simulink model "ramadan_2021"  (R2020a)
settings: Solver=ode15s  StartTime=0.0  StopTime=20  MaxStep=1e-2  MinStep=1e-20  RelTol=1e-3
StartFcn:
  | tic
StopFcn:
  | toc
  | 
  | 
  | %if GimbalLockFlag
  |  % fprintf(2, 'Almost reached Gimbal Lock of IMU. Simulation stopped.\n')
  | %end
  | 
  | %fprintf('Elapsed time: %4.2f sec (%4.2f%% realtime)\n', a, tout(end)/a*100)
values from neighbouring files (symbols this model uses):
  Balance02 = param(28:31)    [assign_parameters.m]
  Balance13 = param(32:35)    [assign_parameters.m]
  BalanceTrunk = param(22:23)    [assign_parameters.m]
  BalanceTrunkLat = param(24:27)    [assign_parameters.m]
  BasisStim = param(1:11)    [assign_parameters.m]
  CompliantLeg = param(12:14)    [assign_parameters.m]
  CompliantLegLat = param(15)    [assign_parameters.m]
  PreventKneeOverextension = param(16:21)    [assign_parameters.m]
  propulsion = dataset(i,3)    [AssignDataset_BasisPoints.m]    (also in assign_parameters.m = param(43))
  stepDur = dataset(i,2)    [AssignDataset_BasisPoints.m]    (also in assign_parameters.m = param(44))
  Target02 = dataset(i,8:10)    [AssignDataset_BasisPoints.m]    (also in assign_parameters.m = param(36:38))
  Target13 = dataset(i,5:7)    [AssignDataset_BasisPoints.m]    (also in assign_parameters.m = param(39:41))
  Target_lat = param(45)    [assign_parameters.m]
  theta0 = dataset(i,4)    [AssignDataset_BasisPoints.m]    (also in assign_parameters.m = param(42))
  v_init = dataset(i,1)    [AssignDataset_BasisPoints.m]    (also in assign_parameters.m = 1.25)
  WramameiSL_1000 = readmatrix('WSL_1000_Norm_Sigmoid_MSE_cont.csv')    [nms3D_prep.m]
  ZramameiSL_1000 = readmatrix('ZSL_1000_Norm_Sigmoid_MSE_cont.csv')    [nms3D_prep.m]
undefined symbols (not defined in the file or in its folder): ICs, mParams, X, Y, Z
libraries: nesl_utility x110, sm_lib x88, simulink x81, eeGeneralControl x30, robotmaniplib x10, dspinverses x9, robotcorelib x5, dspmathops x3, vrlib x1
(part 5 of 8)

== system ramadan_2021/Body and Contact Model/R Leg/Sensor Right Ankle ==
  note: Position and Velocity Sensor in World Frame
  Frame Sensor : sm_lib/Frames and Transforms/Transform Sensor  MeasurementFrame=Base  SenseAngle=off  SenseAxis=off  SenseAngle1=off  SenseAngle2=off  SenseAngle3=off  SenseQ=off  SenseR=off  SenseOmegaX=off  SenseOmegaY=off  SenseOmegaZ=off  SenseOmega1=off  SenseOmega2=off  SenseOmega3=off  SenseQDot=off  SenseRDot=off  SenseAlphaX=off  SenseAlphaY=off  SenseAlphaZ=off  SenseAlpha1=off  SenseAlpha2=off  SenseAlpha3=off  SenseQDDot=off  SenseRDDot=off  SenseX=on  SenseY=on  SenseZ=on  SenseRad=off  SenseAzim=off  SenseDist=off  SenseInc=off  SenseXDot=on  SenseYDot=on  SenseZDot=on  SenseRadDot=off  SenseAzimDot=off  SenseDistDot=off  SenseIncDot=off  SenseXDDot=off  SenseYDDot=off  SenseZDDot=off  SenseRadDDot=off  SenseAzimDDot=off  SenseDistDDot=off  SenseIncDDot=off
  Mux : Mux  Inputs=3
  Mux1 : Mux  Inputs=3
  PS-Simulink Converter1 : nesl_utility/PS-Simulink Converter  PhysicalDomain=network_engine_domain  SubClassName=ps_output  LeftPortType=input  RightPortType=output  PseudoPeriodic=off  Frequencies=[]  Unit=m  AffineConversion=off
  PS-Simulink Converter12 : nesl_utility/PS-Simulink Converter  PhysicalDomain=network_engine_domain  SubClassName=ps_output  LeftPortType=input  RightPortType=output  PseudoPeriodic=off  Frequencies=[]  Unit=m  AffineConversion=off
  PS-Simulink Converter2 : nesl_utility/PS-Simulink Converter  PhysicalDomain=network_engine_domain  SubClassName=ps_output  LeftPortType=input  RightPortType=output  PseudoPeriodic=off  Frequencies=[]  Unit=m  AffineConversion=off
  PS-Simulink Converter3 : nesl_utility/PS-Simulink Converter  PhysicalDomain=network_engine_domain  SubClassName=ps_output  LeftPortType=input  RightPortType=output  PseudoPeriodic=off  Frequencies=[]  Unit=m/s  AffineConversion=off
  PS-Simulink Converter4 : nesl_utility/PS-Simulink Converter  PhysicalDomain=network_engine_domain  SubClassName=ps_output  LeftPortType=input  RightPortType=output  PseudoPeriodic=off  Frequencies=[]  Unit=m/s  AffineConversion=off
  PS-Simulink Converter5 : nesl_utility/PS-Simulink Converter  PhysicalDomain=network_engine_domain  SubClassName=ps_output  LeftPortType=input  RightPortType=output  PseudoPeriodic=off  Frequencies=[]  Unit=m/s  AffineConversion=off
  World Frame : sm_lib/Frames and Transforms/World Frame
  Frame : PMIOPort  Side=Left
  Position [m] : Outport  VectorParamsAs1DForOutWhenUnconnected=off
  Velocity [m/s] : Outport  Port=2  VectorParamsAs1DForOutWhenUnconnected=off
  wires:
  PS-Simulink Converter12/1 -> Mux/1
  PS-Simulink Converter1/1 -> Mux/2
  PS-Simulink Converter2/1 -> Mux/3
  Mux/1 -> Position [m]/1
  PS-Simulink Converter5/1 -> Mux1/3
  PS-Simulink Converter4/1 -> Mux1/1
  Mux1/1 -> Velocity [m/s]/1
  PS-Simulink Converter3/1 -> Mux1/2
  connections:
  Frame Sensor/RConn1 -- Frame/RConn1
  PS-Simulink Converter12/LConn1 -- Frame Sensor/RConn2
  Frame Sensor/RConn3 -- PS-Simulink Converter1/LConn1
  Frame Sensor/RConn4 -- PS-Simulink Converter2/LConn1
  Frame Sensor/RConn7 -- PS-Simulink Converter5/LConn1
  Frame Sensor/RConn5 -- PS-Simulink Converter4/LConn1
  Frame Sensor/RConn6 -- PS-Simulink Converter3/LConn1
  World Frame/RConn1 -- Frame Sensor/LConn1

== system ramadan_2021/Body and Contact Model/R Leg/Shank ==
  Solid : sm_lib/Body Elements/Brick Solid  GraphicAmbientColor=[0.15 0.15 0.15 1.0]  BasedOnType=Density  BrickDimensions="[mParams.bodies.shank.d  mParams.bodies.shank.l mParams.bodies.shank.b]"  BrickDimensionUnits=m  CenterOfMass=mParams.bodies.shank.CG  CenterOfMassUnits=m  GraphicDiffuseColor=[1 0.5 0.5]  Density=2.7  DensityUnits=g/cm^3  DoExposeReferenceFrame=on  GraphicEmissiveColor=[0 0 0 1.0]  ExportEntireGeometry=off  SerializedFrames=<Frames><Frame><Id>Frame1</Id><Value><Name>F1</Name><Origin><Source>CenterOfMassFrame</Source><FeatureName></FeatureName></Origin><PrimaryAxis><DefinedDirection>+Z</DefinedDirection><Source>ReferenceFrame</Source><SourceDirection>+Z</SourceDirection><FeatureName></FeatureName></PrimaryAxis><SecondaryAxis><DefinedDirection>+X</DefinedDirection><Source>ReferenceFrame</Source><SourceDirection>+X</SourceDirection><FeatureName></FeatureName></SecondaryAxis></Value></Frame></Frames>  MarkerShape=Sphere  MarkerSize=10  GraphicType=FromGeometry  InertiaType=Custom  Mass=mParams.bodies.shank.m  MassUnits=kg  MomentsOfInertia=mParams.bodies.shank.In  MomentsOfInertiaUnits=kg*m^2  GraphicOpacity=1.0  ProductsOfInertia=[0 0 0]  ProductsOfInertiaUnits=kg*m^2  GraphicShininess=75  GraphicSpecularColor=[0.5 0.5 0.5 1.0]  GraphicVisPropType=SimpleVisualProperties
  Transform CS1 to MidSegment : sm_lib/Frames and Transforms/Rigid Transform  TranslationMethod=Cartesian  TranslationStandardOffset=0  TranslationLengthUnit=m  TranslationStandardAxis=+Y  TranslationCartesianOffset=[0 -mParams.bodies.shank.l/2 0]  TranslationROffset=0  TranslationROffsetUnits=m  TranslationZOffset=0  TranslationZOffsetUnits=m  TranslationThetaOffset=0  TranslationThetaOffsetUnits=deg  RotationMethod=None  RotationAngleUnits=deg  RotationStandardAxis=+X  RotationAngle=-90  RotationArbitraryAxis=[0 0 1]  FollAlignAxisA=+X  BaseAlignAxisA=+Y  FollAlignAxisB=+Y  BaseAlignAxisB=+Z  RotationSequenceAxes=FollowerAxes  RotationSequence=XYX  RotationSequenceAngles=[0 0 0]  RotationSequenceAnglesUnits=deg  RotationMatrix=[1 0 0; 0 1 0; 0 0 1]
  Transform MidSegment to CS2 : sm_lib/Frames and Transforms/Rigid Transform  TranslationMethod=Cartesian  TranslationStandardOffset=0  TranslationLengthUnit=m  TranslationStandardAxis=+Y  TranslationCartesianOffset=[ 0 -mParams.bodies.shank.l/2 0]  TranslationROffset=0  TranslationROffsetUnits=m  TranslationZOffset=0  TranslationZOffsetUnits=m  TranslationThetaOffset=0  TranslationThetaOffsetUnits=deg  RotationMethod=None  RotationAngleUnits=deg  RotationStandardAxis=+X  RotationAngle=90  RotationArbitraryAxis=[0 0 1]  FollAlignAxisA=+X  BaseAlignAxisA=+Y  FollAlignAxisB=+Y  BaseAlignAxisB=+Z  RotationSequenceAxes=FollowerAxes  RotationSequence=XYX  RotationSequenceAngles=[0 0 0]  RotationSequenceAnglesUnits=deg  RotationMatrix=[1 0 0; 0 1 0; 0 0 1]
  CS1 : PMIOPort  Side=Left
  CS2 : PMIOPort  Port=2  Side=Right
  connections:
  Transform MidSegment to CS2/LConn1 -- Transform CS1 to MidSegment/RConn1 -- Solid/RConn1
  Transform CS1 to MidSegment/LConn1 -- CS1/RConn1
  Transform MidSegment to CS2/RConn1 -- CS2/RConn1

== system ramadan_2021/Body and Contact Model/R Leg/Thigh ==
  Solid1 : sm_lib/Body Elements/Brick Solid  GraphicAmbientColor=[0.15 0.15 0.15 1.0]  BasedOnType=Density  BrickDimensions=[mParams.bodies.thigh.d mParams.bodies.thigh.l mParams.bodies.thigh.b]  BrickDimensionUnits=m  CenterOfMass=mParams.bodies.thigh.CG  CenterOfMassUnits=m  GraphicDiffuseColor=[1 0.5 0.5]  Density=2.7  DensityUnits=g/cm^3  DoExposeReferenceFrame=on  GraphicEmissiveColor=[0 0 0 1.0]  ExportEntireGeometry=off  SerializedFrames=<Frames><Frame><Id>Frame1</Id><Value><Name>F1</Name><Origin><Source>CenterOfMassFrame</Source><FeatureName></FeatureName></Origin><PrimaryAxis><DefinedDirection>+Z</DefinedDirection><Source>ReferenceFrame</Source><SourceDirection>+Z</SourceDirection><FeatureName></FeatureName></PrimaryAxis><SecondaryAxis><DefinedDirection>+X</DefinedDirection><Source>ReferenceFrame</Source><SourceDirection>+X</SourceDirection><FeatureName></FeatureName></SecondaryAxis></Value></Frame></Frames>  MarkerShape=Sphere  MarkerSize=10  GraphicType=FromGeometry  InertiaType=Custom  Mass=mParams.bodies.thigh.m  MassUnits=kg  MomentsOfInertia=mParams.bodies.thigh.In  MomentsOfInertiaUnits=kg*m^2  GraphicOpacity=1.0  ProductsOfInertia=[0 0 0]  ProductsOfInertiaUnits=kg*m^2  GraphicShininess=75  GraphicSpecularColor=[0.5 0.5 0.5 1.0]  GraphicVisPropType=SimpleVisualProperties
  Transform CG to MidSegment : sm_lib/Frames and Transforms/Rigid Transform  TranslationMethod=Cartesian  TranslationStandardOffset=0  TranslationLengthUnit=m  TranslationStandardAxis=+Y  TranslationCartesianOffset=[0 -mParams.bodies.thigh.l/2 0]  TranslationROffset=0  TranslationROffsetUnits=m  TranslationZOffset=0  TranslationZOffsetUnits=m  TranslationThetaOffset=0  TranslationThetaOffsetUnits=deg  RotationMethod=None  RotationAngleUnits=deg  RotationStandardAxis=+X  RotationAngle=90  RotationArbitraryAxis=[0 0 1]  FollAlignAxisA=+X  BaseAlignAxisA=+Y  FollAlignAxisB=+Y  BaseAlignAxisB=+Z  RotationSequenceAxes=FollowerAxes  RotationSequence=XYX  RotationSequenceAngles=[0 0 0]  RotationSequenceAnglesUnits=deg  RotationMatrix=[1 0 0; 0 1 0; 0 0 1]
  Transform CS1 to MidSegment : sm_lib/Frames and Transforms/Rigid Transform  TranslationMethod=Cartesian  TranslationStandardOffset=0  TranslationLengthUnit=m  TranslationStandardAxis=+Y  TranslationCartesianOffset=[0 -mParams.bodies.thigh.l/2 0]  TranslationROffset=0  TranslationROffsetUnits=m  TranslationZOffset=0  TranslationZOffsetUnits=m  TranslationThetaOffset=0  TranslationThetaOffsetUnits=deg  RotationMethod=None  RotationAngleUnits=deg  RotationStandardAxis=+X  RotationAngle=-90  RotationArbitraryAxis=[0 0 1]  FollAlignAxisA=+X  BaseAlignAxisA=+Y  FollAlignAxisB=+Y  BaseAlignAxisB=+Z  RotationSequenceAxes=FollowerAxes  RotationSequence=XYX  RotationSequenceAngles=[0 0 0]  RotationSequenceAnglesUnits=deg  RotationMatrix=[1 0 0; 0 1 0; 0 0 1]
  CS1 : PMIOPort  Side=Left
  CS2 : PMIOPort  Port=2  Side=Right
  connections:
  Transform CG to MidSegment/LConn1 -- Solid1/RConn1 -- Transform CS1 to MidSegment/RConn1
  Transform CS1 to MidSegment/LConn1 -- CS1/RConn1
  Transform CG to MidSegment/RConn1 -- CS2/RConn1

== system ramadan_2021/Body and Contact Model/Vestibular System/  XYZ Sensor Left Hip ==
  note: Simplified IMU Model
  Frame Sensor : sm_lib/Frames and Transforms/Transform Sensor  MeasurementFrame=World  SenseAngle=off  SenseAxis=off  SenseAngle1=off  SenseAngle2=off  SenseAngle3=off  SenseQ=off  SenseR=off  SenseOmegaX=off  SenseOmegaY=off  SenseOmegaZ=off  SenseOmega1=off  SenseOmega2=off  SenseOmega3=off  SenseQDot=off  SenseRDot=off  SenseAlphaX=off  SenseAlphaY=off  SenseAlphaZ=off  SenseAlpha1=off  SenseAlpha2=off  SenseAlpha3=off  SenseQDDot=off  SenseRDDot=off  SenseX=on  SenseY=on  SenseZ=on  SenseRad=off  SenseAzim=off  SenseDist=off  SenseInc=off  SenseXDot=on  SenseYDot=on  SenseZDot=on  SenseRadDot=off  SenseAzimDot=off  SenseDistDot=off  SenseIncDot=off  SenseXDDot=off  SenseYDDot=off  SenseZDDot=off  SenseRadDDot=off  SenseAzimDDot=off  SenseDistDDot=off  SenseIncDDot=off
  Mux1 : Mux  Inputs=3
  Mux3 : Mux  Inputs=3
  PS-Simulink Converter : nesl_utility/PS-Simulink Converter  PhysicalDomain=network_engine_domain  SubClassName=ps_output  LeftPortType=input  RightPortType=output  PseudoPeriodic=off  Frequencies=[]  Unit=m  AffineConversion=off
  PS-Simulink Converter1 : nesl_utility/PS-Simulink Converter  PhysicalDomain=network_engine_domain  SubClassName=ps_output  LeftPortType=input  RightPortType=output  PseudoPeriodic=off  Frequencies=[]  Unit=m  AffineConversion=off
  PS-Simulink Converter2 : nesl_utility/PS-Simulink Converter  PhysicalDomain=network_engine_domain  SubClassName=ps_output  LeftPortType=input  RightPortType=output  PseudoPeriodic=off  Frequencies=[]  Unit=m/s  AffineConversion=off
  PS-Simulink Converter3 : nesl_utility/PS-Simulink Converter  PhysicalDomain=network_engine_domain  SubClassName=ps_output  LeftPortType=input  RightPortType=output  PseudoPeriodic=off  Frequencies=[]  Unit=m/s  AffineConversion=off
  PS-Simulink Converter4 : nesl_utility/PS-Simulink Converter  PhysicalDomain=network_engine_domain  SubClassName=ps_output  LeftPortType=input  RightPortType=output  PseudoPeriodic=off  Frequencies=[]  Unit=m  AffineConversion=off
  PS-Simulink Converter5 : nesl_utility/PS-Simulink Converter  PhysicalDomain=network_engine_domain  SubClassName=ps_output  LeftPortType=input  RightPortType=output  PseudoPeriodic=off  Frequencies=[]  Unit=m/s  AffineConversion=off
  World Frame : sm_lib/Frames and Transforms/World Frame
  frame : PMIOPort  Side=Left
  Hip Position [m] : Outport  VectorParamsAs1DForOutWhenUnconnected=off
  Hip Velocity [m/s] : Outport  Port=2  VectorParamsAs1DForOutWhenUnconnected=off
  wires:
  PS-Simulink Converter4/1 -> Mux3/3
  PS-Simulink Converter/1 -> Mux3/1
  Mux3/1 -> Hip Position [m]/1
  PS-Simulink Converter1/1 -> Mux3/2
  PS-Simulink Converter3/1 -> Mux1/2
  PS-Simulink Converter5/1 -> Mux1/3
  PS-Simulink Converter2/1 -> Mux1/1
  Mux1/1 -> Hip Velocity [m/s]/1
  connections:
  Frame Sensor/RConn1 -- frame/RConn1
  World Frame/RConn1 -- Frame Sensor/LConn1
  Frame Sensor/RConn4 -- PS-Simulink Converter4/LConn1
  Frame Sensor/RConn3 -- PS-Simulink Converter1/LConn1
  Frame Sensor/RConn2 -- PS-Simulink Converter/LConn1
  Frame Sensor/RConn5 -- PS-Simulink Converter2/LConn1
  Frame Sensor/RConn6 -- PS-Simulink Converter3/LConn1
  Frame Sensor/RConn7 -- PS-Simulink Converter5/LConn1

== system ramadan_2021/Body and Contact Model/Vestibular System/  XYZ Sensor Right Hip ==
  note: Simplified IMU Model
  Frame Sensor : sm_lib/Frames and Transforms/Transform Sensor  MeasurementFrame=World  SenseAngle=off  SenseAxis=off  SenseAngle1=off  SenseAngle2=off  SenseAngle3=off  SenseQ=off  SenseR=off  SenseOmegaX=off  SenseOmegaY=off  SenseOmegaZ=off  SenseOmega1=off  SenseOmega2=off  SenseOmega3=off  SenseQDot=off  SenseRDot=off  SenseAlphaX=off  SenseAlphaY=off  SenseAlphaZ=off  SenseAlpha1=off  SenseAlpha2=off  SenseAlpha3=off  SenseQDDot=off  SenseRDDot=off  SenseX=on  SenseY=on  SenseZ=on  SenseRad=off  SenseAzim=off  SenseDist=off  SenseInc=off  SenseXDot=on  SenseYDot=on  SenseZDot=on  SenseRadDot=off  SenseAzimDot=off  SenseDistDot=off  SenseIncDot=off  SenseXDDot=off  SenseYDDot=off  SenseZDDot=off  SenseRadDDot=off  SenseAzimDDot=off  SenseDistDDot=off  SenseIncDDot=off
  Mux1 : Mux  Inputs=3
  Mux3 : Mux  Inputs=3
  PS-Simulink Converter : nesl_utility/PS-Simulink Converter  PhysicalDomain=network_engine_domain  SubClassName=ps_output  LeftPortType=input  RightPortType=output  PseudoPeriodic=off  Frequencies=[]  Unit=m  AffineConversion=off
  PS-Simulink Converter1 : nesl_utility/PS-Simulink Converter  PhysicalDomain=network_engine_domain  SubClassName=ps_output  LeftPortType=input  RightPortType=output  PseudoPeriodic=off  Frequencies=[]  Unit=m  AffineConversion=off
  PS-Simulink Converter2 : nesl_utility/PS-Simulink Converter  PhysicalDomain=network_engine_domain  SubClassName=ps_output  LeftPortType=input  RightPortType=output  PseudoPeriodic=off  Frequencies=[]  Unit=m/s  AffineConversion=off
  PS-Simulink Converter3 : nesl_utility/PS-Simulink Converter  PhysicalDomain=network_engine_domain  SubClassName=ps_output  LeftPortType=input  RightPortType=output  PseudoPeriodic=off  Frequencies=[]  Unit=m/s  AffineConversion=off
  PS-Simulink Converter4 : nesl_utility/PS-Simulink Converter  PhysicalDomain=network_engine_domain  SubClassName=ps_output  LeftPortType=input  RightPortType=output  PseudoPeriodic=off  Frequencies=[]  Unit=m  AffineConversion=off
  PS-Simulink Converter5 : nesl_utility/PS-Simulink Converter  PhysicalDomain=network_engine_domain  SubClassName=ps_output  LeftPortType=input  RightPortType=output  PseudoPeriodic=off  Frequencies=[]  Unit=m/s  AffineConversion=off
  World Frame : sm_lib/Frames and Transforms/World Frame
  frame : PMIOPort  Side=Left
  Hip Position [m] : Outport  VectorParamsAs1DForOutWhenUnconnected=off
  Hip Velocity [m/s] : Outport  Port=2  VectorParamsAs1DForOutWhenUnconnected=off
  wires:
  PS-Simulink Converter4/1 -> Mux3/3
  PS-Simulink Converter/1 -> Mux3/1
  Mux3/1 -> Hip Position [m]/1
  PS-Simulink Converter1/1 -> Mux3/2
  PS-Simulink Converter3/1 -> Mux1/2
  PS-Simulink Converter5/1 -> Mux1/3
  PS-Simulink Converter2/1 -> Mux1/1
  Mux1/1 -> Hip Velocity [m/s]/1
  connections:
  Frame Sensor/RConn1 -- frame/RConn1
  World Frame/RConn1 -- Frame Sensor/LConn1
  Frame Sensor/RConn4 -- PS-Simulink Converter4/LConn1
  Frame Sensor/RConn3 -- PS-Simulink Converter1/LConn1
  Frame Sensor/RConn2 -- PS-Simulink Converter/LConn1
  Frame Sensor/RConn5 -- PS-Simulink Converter2/LConn1
  Frame Sensor/RConn6 -- PS-Simulink Converter3/LConn1
  Frame Sensor/RConn7 -- PS-Simulink Converter5/LConn1

== system ramadan_2021/Body and Contact Model/Vestibular System/Align Axis ==
  note: Axis Alignment: We rotate the position vectors in the frame of the moving direction (R). For the lateral rotation, we measure the rotation of line that connects the two hip positions in the (0,0,1)-axis. For the saggital rotation, we measure the rotation of the line between Trunk-CoM (x,y,0) and the average position of the two hip joints (Hr+Hl)/2 in the (0,1,0)-axis
  Ankle Position Right [m] : Inport
  Ankle Position Left [m] : Inport  Port=2
  "R " : Inport  Port=3
  Position Trunk [m] : Inport  Port=4
  Velocity Trunk [m/s] : Inport  Port=5
  Hip Position Left [m] : Inport  Port=6
  Hip Position Right [m] : Inport  Port=7
  Compute Lateral Rotation : Subsystem
  Compute Saggital Rotation : Subsystem
  Filtered Derivative (Discrete or Continuous) : eeGeneralControl/Filtered Derivative (Discrete or Continuous)  K=1  T=mParams.control.delays.longloop/2  B=inf  A=-inf  minRatio=10  init_option=Inherited from block input  x0=0  Ts=0
      settings: SourceProductBaseCode=PS
  Filtered Derivative (Discrete or Continuous)1 : eeGeneralControl/Filtered Derivative (Discrete or Continuous)  K=1  T=mParams.control.delays.longloop/2  B=inf  A=-inf  minRatio=10  init_option=Inherited from block input  x0=0  Ts=0
      settings: SourceProductBaseCode=PS
  Matrix Multiply{,1..4,6..8} (8 alike) : Product  Multiplication=Matrix(*)
  Minus{1..3,15} (4 alike) : Sum  Inputs=+-
  Ankle Position Left (body frame) : Outport
  Ankle Position Right (body frame) : Outport  Port=2
  Trunk Velocity (body frame) : Outport  Port=3
  Saggital Trunk Rotation [rad] (body frame) : Outport  Port=4
  Lateral Trunk Rotation [rad] (body frame) : Outport  Port=5
  Saggital Trunk Rotation Velocity [rad/s] (body frame) : Outport  Port=6
  Lateral Trunk Rotation Velocity [rad/s] (body frame) : Outport  Port=7
  Heel Position Left (body frame) : Outport  Port=8
  Heel Position Right (body frame) : Outport  Port=9
  wires:
  Minus15/1 -> Matrix Multiply1/2
  Ankle Position Left [m]/1 -> Minus2/2
  Ankle Position Right [m]/1 -> Minus15/2
  Matrix Multiply/1 -> Ankle Position Left (body frame)/1
  Minus2/1 -> Matrix Multiply/2
  Matrix Multiply1/1 -> Ankle Position Right (body frame)/1
  Velocity Trunk [m/s]/1 -> Matrix Multiply2/2
  Matrix Multiply2/1 -> Trunk Velocity (body frame)/1
  Hip Position Right [m]/1 -> Matrix Multiply6/2
  Hip Position Left [m]/1 -> Matrix Multiply7/2
  Compute Lateral Rotation/1(Lateral Rotation) -> Lateral Trunk Rotation [rad] (body frame)/1, Filtered Derivative (Discrete or Continuous)1/1
  Matrix Multiply7/1 -> Compute Saggital Rotation/1(Hip Position Left [m]), Compute Lateral Rotation/1(Hip Left)
  Matrix Multiply6/1 -> Compute Saggital Rotation/2(Hip Position Right [m]), Compute Lateral Rotation/2(Hip Right)
  Compute Saggital Rotation/1(Saggital Rotation) -> Saggital Trunk Rotation [rad] (body frame)/1, Filtered Derivative (Discrete or Continuous)/1
  Matrix Multiply8/1 -> Compute Saggital Rotation/3(Trunk Position [m])
  Filtered Derivative (Discrete or Continuous)1/1 -> Lateral Trunk Rotation Velocity [rad/s] (body frame)/1
  Filtered Derivative (Discrete or Continuous)/1 -> Saggital Trunk Rotation Velocity [rad/s] (body frame)/1
  [LHL] -> Minus1/2
  Minus1/1 -> Matrix Multiply3/2
  Matrix Multiply3/1 -> Heel Position Left (body frame)/1
  Matrix Multiply4/1 -> Heel Position Right (body frame)/1
  Minus3/1 -> Matrix Multiply4/2
  [LHR] -> Minus3/2
  Position Trunk [m]/1 -> Minus3/1, Minus1/1, Minus15/1, Matrix Multiply8/2, Minus2/1
  "R "/1 -> Matrix Multiply4/1, Matrix Multiply3/1, Matrix Multiply8/1, Matrix Multiply6/1, Matrix Multiply7/1, Matrix Multiply2/1, Matrix Multiply1/1, Matrix Multiply/1

== system ramadan_2021/Body and Contact Model/Vestibular System/R Movement direction ==
  Hip Right : Inport
  Hip Left : Inport  Port=2
  Constant : Constant  Value=[0;1;0]
  Cross Product : vrlib/Utilities/Cross Product
  Gain : Gain  Gain=[1 0 1]
  Gain1 : Gain  Gain=[1 0 1]
  Matrix Concatenate : Concatenate  NumInputs=3  Mode=Multidimensional array  ConcatenateDimension=2
  Minus : Sum  Inputs=+-
  Normalization : dspmathops/Normalization  NormType=2-norm  Bias=1e-10  NormOver=Each column  Dimension=1  roundingMode=Floor  overflowMode=off  accumDataTypeStr=Inherit: Same as product output  accumLastDataTypeStr=Inherit: Same as product output  outputDataTypeStr=Inherit: Same as product output  outputMin=[]  outputMax=[]  outputLastDataTypeStr=Inherit: Same as product output
  Transpose : Math  Operator=transpose  SaturateOnIntegerOverflow=on
  "R " : Outport
  wires:
  Constant/1 -> Matrix Concatenate/2, Cross Product/1
  Normalization/1 -> Matrix Concatenate/3, Cross Product/2
  Hip Right/1 -> Gain/1
  Hip Left/1 -> Gain1/1
  Minus/1 -> Normalization/1
  Matrix Concatenate/1 -> Transpose/1
  Transpose/1 -> "R "/1
  Cross Product/1 -> Matrix Concatenate/1
  Gain/1 -> Minus/1
  Gain1/1 -> Minus/2

== system ramadan_2021/Body and Contact Model/Vestibular System/Trunk Sensor  ==
  Coordinate Transformation Conversion1 : robotcorelib/Coordinate Transformation Conversion  InputRepresentation=Quaternion  InputEulerSequence=ZYX  ShowTrVecInputPort=on  OutputRepresentation=Euler Angles  OutputEulerSequence=XYZ  ShowTrVecOutputPort=on  SimulateUsing=Code generation
      settings: SourceProductBaseCode=NV,RO,RR
  Frame Sensor : sm_lib/Frames and Transforms/Transform Sensor  MeasurementFrame=World  SenseAngle=off  SenseAxis=off  SenseAngle1=off  SenseAngle2=off  SenseAngle3=off  SenseQ=on  SenseR=off  SenseOmegaX=on  SenseOmegaY=on  SenseOmegaZ=on  SenseOmega1=off  SenseOmega2=off  SenseOmega3=off  SenseQDot=off  SenseRDot=off  SenseAlphaX=off  SenseAlphaY=off  SenseAlphaZ=off  SenseAlpha1=off  SenseAlpha2=off  SenseAlpha3=off  SenseQDDot=off  SenseRDDot=off  SenseX=on  SenseY=on  SenseZ=on  SenseRad=off  SenseAzim=off  SenseDist=off  SenseInc=off  SenseXDot=on  SenseYDot=on  SenseZDot=on  SenseRadDot=off  SenseAzimDot=off  SenseDistDot=off  SenseIncDot=off  SenseXDDot=off  SenseYDDot=off  SenseZDDot=off  SenseRadDDot=off  SenseAzimDDot=off  SenseDistDDot=off  SenseIncDDot=off
  Mux2 : Mux  Inputs=3
  Mux3 : Mux  Inputs=3
  Mux4 : Mux  Inputs=3
  PS-Simulink Converter : nesl_utility/PS-Simulink Converter  PhysicalDomain=network_engine_domain  SubClassName=ps_output  LeftPortType=input  RightPortType=output  PseudoPeriodic=off  Frequencies=[]  Unit=m  AffineConversion=off
  PS-Simulink Converter1 : nesl_utility/PS-Simulink Converter  PhysicalDomain=network_engine_domain  SubClassName=ps_output  LeftPortType=input  RightPortType=output  PseudoPeriodic=off  Frequencies=[]  Unit=m  AffineConversion=off
  PS-Simulink Converter10 : nesl_utility/PS-Simulink Converter  PhysicalDomain=network_engine_domain  SubClassName=ps_output  LeftPortType=input  RightPortType=output  PseudoPeriodic=off  Frequencies=[]  Unit=rad/s  AffineConversion=off
  PS-Simulink Converter11 : nesl_utility/PS-Simulink Converter  PhysicalDomain=network_engine_domain  SubClassName=ps_output  LeftPortType=input  RightPortType=output  PseudoPeriodic=off  Frequencies=[]  Unit=rad/s  AffineConversion=off
  PS-Simulink Converter12 : nesl_utility/PS-Simulink Converter  PhysicalDomain=network_engine_domain  SubClassName=ps_output  LeftPortType=input  RightPortType=output  PseudoPeriodic=off  Frequencies=[]  Unit=1  AffineConversion=off
  PS-Simulink Converter2 : nesl_utility/PS-Simulink Converter  PhysicalDomain=network_engine_domain  SubClassName=ps_output  LeftPortType=input  RightPortType=output  PseudoPeriodic=off  Frequencies=[]  Unit=m/s  AffineConversion=off
  PS-Simulink Converter3 : nesl_utility/PS-Simulink Converter  PhysicalDomain=network_engine_domain  SubClassName=ps_output  LeftPortType=input  RightPortType=output  PseudoPeriodic=off  Frequencies=[]  Unit=m/s  AffineConversion=off
  PS-Simulink Converter4 : nesl_utility/PS-Simulink Converter  PhysicalDomain=network_engine_domain  SubClassName=ps_output  LeftPortType=input  RightPortType=output  PseudoPeriodic=off  Frequencies=[]  Unit=m  AffineConversion=off
  PS-Simulink Converter5 : nesl_utility/PS-Simulink Converter  PhysicalDomain=network_engine_domain  SubClassName=ps_output  LeftPortType=input  RightPortType=output  PseudoPeriodic=off  Frequencies=[]  Unit=m/s  AffineConversion=off
  PS-Simulink Converter9 : nesl_utility/PS-Simulink Converter  PhysicalDomain=network_engine_domain  SubClassName=ps_output  LeftPortType=input  RightPortType=output  PseudoPeriodic=off  Frequencies=[]  Unit=rad/s  AffineConversion=off
  World Frame : sm_lib/Frames and Transforms/World Frame
  frame : PMIOPort  Side=Left
  Position Trunk [m] : Outport  VectorParamsAs1DForOutWhenUnconnected=off
  Velocity Trunk [m/s] : Outport  Port=2  VectorParamsAs1DForOutWhenUnconnected=off
  Rotation Velocity Trunk [rad/s] : Outport  Port=3  VectorParamsAs1DForOutWhenUnconnected=off
  Rotation Trunk [rad] : Outport  Port=4  VectorParamsAs1DForOutWhenUnconnected=off
  wires:
  PS-Simulink Converter4/1 -> Mux3/3
  PS-Simulink Converter3/1 -> Mux4/2
  PS-Simulink Converter5/1 -> Mux4/3
  PS-Simulink Converter/1 -> Mux3/1
  Mux3/1 -> Position Trunk [m]/1
  Mux4/1 -> Velocity Trunk [m/s]/1
  PS-Simulink Converter2/1 -> Mux4/1
  PS-Simulink Converter1/1 -> Mux3/2
  PS-Simulink Converter9/1 -> Mux2/1
  Mux2/1 -> Rotation Velocity Trunk [rad/s]/1
  PS-Simulink Converter11/1 -> Mux2/3
  PS-Simulink Converter10/1 -> Mux2/2
  PS-Simulink Converter12/1 -> Coordinate Transformation Conversion1/1
  Coordinate Transformation Conversion1/1 -> Rotation Trunk [rad]/1
  connections:
  Frame Sensor/RConn1 -- frame/RConn1
  World Frame/RConn1 -- Frame Sensor/LConn1
  Frame Sensor/RConn11 -- PS-Simulink Converter5/LConn1
  Frame Sensor/RConn10 -- PS-Simulink Converter3/LConn1
  Frame Sensor/RConn9 -- PS-Simulink Converter2/LConn1
  Frame Sensor/RConn8 -- PS-Simulink Converter4/LConn1
  Frame Sensor/RConn7 -- PS-Simulink Converter1/LConn1
  Frame Sensor/RConn6 -- PS-Simulink Converter/LConn1
  Frame Sensor/RConn5 -- PS-Simulink Converter11/LConn1
  Frame Sensor/RConn4 -- PS-Simulink Converter10/LConn1
  Frame Sensor/RConn3 -- PS-Simulink Converter9/LConn1
  PS-Simulink Converter12/LConn1 -- Frame Sensor/RConn2

== system ramadan_2021/CMA Data/Step Counter/count steps1 ==
  nStep-1 : Inport  LatchByDelayingOutsideSignal=on
  Trigger : TriggerPort  VariantControl=(inherit)  ZeroCross=off
  Constant : Constant
  Sum : Sum  Inputs=|++
  nStep : Outport  InitialOutput=0  VectorParamsAs1DForOutWhenUnconnected=off
  wires:
  Constant/1 -> Sum/2
  nStep-1/1 -> Sum/1
  Sum/1 -> nStep/1

== system ramadan_2021/CMA Data/Step Counter/count steps2 ==
  nStep-1 : Inport  LatchByDelayingOutsideSignal=on
  Trigger : TriggerPort  VariantControl=(inherit)  ZeroCross=off
  Constant : Constant
  Sum : Sum  Inputs=|++
  nStep : Outport  InitialOutput=0  VectorParamsAs1DForOutWhenUnconnected=off
  wires:
  Constant/1 -> Sum/2
  nStep-1/1 -> Sum/1
  Sum/1 -> nStep/1

== system ramadan_2021/CMA Data/check steady state/even ==
  In1 : Inport
  Trigger : TriggerPort  TriggerType=falling  VariantControl=(inherit)  ZeroCross=off
  Out1 : Outport  VectorParamsAs1DForOutWhenUnconnected=off
  wires:
  In1/1 -> Out1/1

== system ramadan_2021/CMA Data/check steady state/odd ==
  In1 : Inport
  Trigger : TriggerPort  VariantControl=(inherit)  ZeroCross=off
  Out1 : Outport  VectorParamsAs1DForOutWhenUnconnected=off
  wires:
  In1/1 -> Out1/1

== system ramadan_2021/Muscle Actuation Layer/Muscles Left/Muscle Dynamics (Vectorized)1 ==
  note: Excitation Contraction Coupling
  note: VECTORIZED Muscle-Tendon Dynamics
  lmtc [m] : Inport
  STIM : Inport  Port=2
  1 : Product  Inputs=**  InputSameDT=on  SaturateOnIntegerOverflow=on  OutDataTypeStr=Inherit: Same as first input
  1./lopt : Gain  Gain=1./mParams.muscles.loptVec  SaturateOnIntegerOverflow=on  OutDataTypeStr=Inherit: Same as input  ParamDataTypeStr=Inherit: Same as input
  1./lopt2 : Gain  Gain=1/mParams.muscles.tauA  SaturateOnIntegerOverflow=on  OutDataTypeStr=Inherit: Same as input  ParamDataTypeStr=Inherit: Same as input
  1/lslack : Gain  Gain=1./mParams.muscles.lslackVec  SaturateOnIntegerOverflow=on  OutDataTypeStr=Inherit: Same as input  ParamDataTypeStr=Inherit: Same as input
  BE force-length relation : Subsystem
  CE force-length relation : Subsystem
  CE inverse force-velocity relation : Subsystem
  Constant : Constant  Value=mParams.muscles.lslackVec
  Fmax : Gain  Gain=mParams.muscles.FmaxVec  SaturateOnIntegerOverflow=on  OutDataTypeStr=Inherit: Same as input  ParamDataTypeStr=Inherit: Same as input
  Fv = Fse / (A*Fce) : Product  Inputs=*/  InputSameDT=on  SaturateOnIntegerOverflow=on  OutDataTypeStr=Inherit: Same as first input
  Integrator : Integrator  InitialConditionSource=external  LowerSaturationLimit=0.05
  Integrator1 : Integrator  InitialConditionSource=external  LowerSaturationLimit=0.05
  PE force-length relation : Subsystem
  SE force-length relation : Subsystem
  Sum : Sum  Inputs=|+-  InputSameDT=on  SaturateOnIntegerOverflow=on  OutDataTypeStr=Inherit: Same as first input
  Sum1 : Sum  Inputs=|+-  InputSameDT=on  SaturateOnIntegerOverflow=on  OutDataTypeStr=Inherit: Same as first input
  Sum2 : Sum  Inputs=|-+  InputSameDT=on  SaturateOnIntegerOverflow=on  OutDataTypeStr=Inherit: Same as first input
  Sum3 : Sum  Inputs=+++  InputSameDT=on  SaturateOnIntegerOverflow=on  OutDataTypeStr=Inherit: Same as first input
  Sum4 : Sum  InputSameDT=on  SaturateOnIntegerOverflow=on  OutDataTypeStr=Inherit: Same as first input
  avoid div by 0 : Constant  Value=eps
  preA : Constant  Value=mParams.muscles.preA
  vmax*lopt : Gain  Gain=mParams.muscles.vmaxVec  SaturateOnIntegerOverflow=on  OutDataTypeStr=Inherit: Same as input  ParamDataTypeStr=Inherit: Same as input
  Fmtc : Outport  InitialOutput=0  VectorParamsAs1DForOutWhenUnconnected=off
  Lce : Outport  Port=2  InitialOutput=0  VectorParamsAs1DForOutWhenUnconnected=off
  Vce : Outport  Port=3  InitialOutput=0  VectorParamsAs1DForOutWhenUnconnected=off
  A : Outport  Port=4  InitialOutput=0  VectorParamsAs1DForOutWhenUnconnected=off
  ForceLengthFactor : Outport  Port=5  VectorParamsAs1DForOutWhenUnconnected=off
  tag scope: fl_L=global, fv_L=global
  wires:
  1./lopt2/1 -> Integrator1/1
  Sum1/1 -> 1./lopt2/1
  CE inverse force-velocity relation/1(v[vmax]) -> vmax*lopt/1
  Fv = Fse / (A*Fce)/1 -> CE inverse force-velocity relation/1(Fv[Fmax]), [fv_L]  "fv"
  Sum3/1 -> Fv = Fse / (A*Fce)/2
  Sum4/1 -> Fv = Fse / (A*Fce)/1
  SE force-length relation/1(fse [Fmax]) -> Fmax/1, Sum4/1
  Integrator1/1 -> Sum1/2, A/1, 1/2
  Fmax/1 -> Fmtc/1  "Fmtc"
  lmtc [m]/1 -> Sum/1, Sum2/2  "lmtc"
  vmax*lopt/1 -> Integrator/1, Vce/1  "vce"
  1./lopt/1 -> CE force-length relation/1(lce [lopt]), BE force-length relation/1(lce [lopt]), PE force-length relation/1(lce [lopt])
  Integrator/1 -> 1./lopt/1, Sum/2, Lce/1  "lce"
  1/1 -> Sum3/3
  1/lslack/1 -> SE force-length relation/1(lse [lslack])
  STIM/1 -> Sum1/1
  Sum/1 -> 1/lslack/1  "lse"
  Constant/1 -> Sum2/1
  PE force-length relation/1(fpe [Fmax]) -> Sum3/1
  BE force-length relation/1(fbe [Fmax]) -> Sum4/2
  avoid div by 0/1 -> Sum3/2
  preA/1 -> Integrator1/2
  Sum2/1 -> Integrator/2
  CE force-length relation/1(fce [Fmax]) -> [fl_L], ForceLengthFactor/1, 1/1

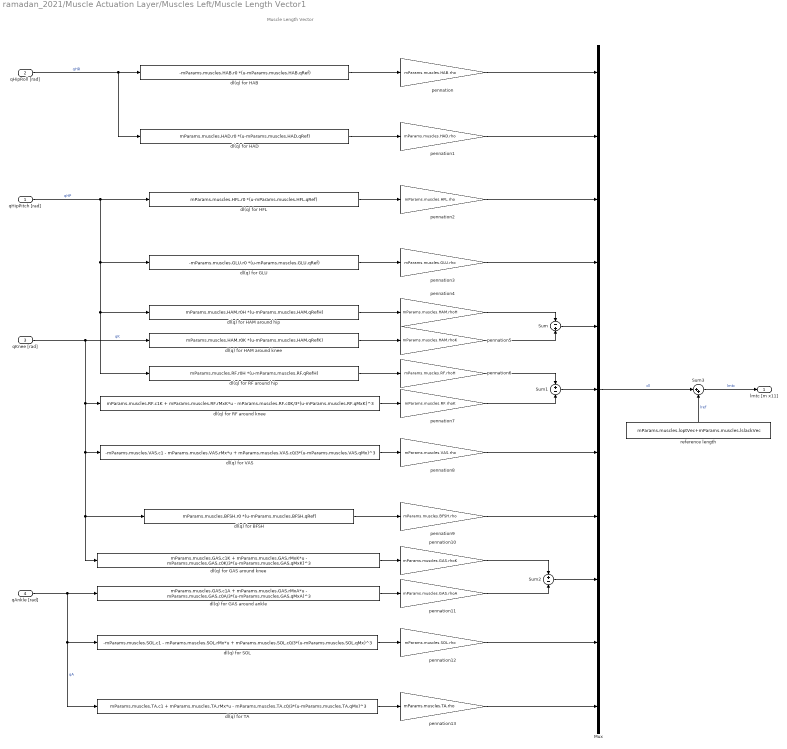
== system ramadan_2021/Muscle Actuation Layer/Muscles Left/Muscle Length Vector1 ==
  note: Muscle Length Vector
  qHipPitch [rad] : Inport
  qHipRoll [rad] : Inport  Port=2
  qKnee [rad] : Inport  Port=3
  qAnkle [rad] : Inport  Port=4
  Mux : Mux  Inputs=11
  Sum : Sum  Inputs=-+
  Sum1 : Sum  Inputs=+-
  Sum2 : Sum  Inputs=+-
  Sum3 : Sum  Inputs=|++
  dl(q) for BFSH : Fcn  Expr=mParams.muscles.BFSH.r0 *(u-mParams.muscles.BFSH.qRef)
  dl(q) for GAS around ankle : Fcn  Expr=mParams.muscles.GAS.c1A + mParams.muscles.GAS.rMxA*u - mParams.muscles.GAS.c0A/3*(u-mParams.muscles.GAS.qMxA)^3
  dl(q) for GAS around knee : Fcn  Expr=mParams.muscles.GAS.c1K + mParams.muscles.GAS.rMxK*u - mParams.muscles.GAS.c0K/3*(u-mParams.muscles.GAS.qMxK)^3
  dl(q) for GLU : Fcn  Expr=-mParams.muscles.GLU.r0 *(u-mParams.muscles.GLU.qRef)
  dl(q) for HAB : Fcn  Expr=-mParams.muscles.HAB.r0 *(u-mParams.muscles.HAB.qRef)
  dl(q) for HAD : Fcn  Expr=mParams.muscles.HAD.r0 *(u-mParams.muscles.HAD.qRef)
  dl(q) for HAM around hip : Fcn  Expr=mParams.muscles.HAM.r0H *(u-mParams.muscles.HAM.qRefH)
  dl(q) for HAM around knee : Fcn  Expr=mParams.muscles.HAM.r0K *(u-mParams.muscles.HAM.qRefK)
  dl(q) for HFL : Fcn  Expr=mParams.muscles.HFL.r0 *(u-mParams.muscles.HFL.qRef)
  dl(q) for RF around hip : Fcn  Expr=mParams.muscles.RF.r0H *(u-mParams.muscles.RF.qRefH)
  dl(q) for RF around knee : Fcn  Expr=mParams.muscles.RF.c1K + mParams.muscles.RF.rMxK*u - mParams.muscles.RF.c0K/3*(u-mParams.muscles.RF.qMxK)^3
  dl(q) for SOL : Fcn  Expr=-mParams.muscles.SOL.c1 - mParams.muscles.SOL.rMx*u + mParams.muscles.SOL.c0/3*(u-mParams.muscles.SOL.qMx)^3
  dl(q) for TA : Fcn  Expr=mParams.muscles.TA.c1 + mParams.muscles.TA.rMx*u - mParams.muscles.TA.c0/3*(u-mParams.muscles.TA.qMx)^3
  dl(q) for VAS : Fcn  Expr=-mParams.muscles.VAS.c1 - mParams.muscles.VAS.rMx*u + mParams.muscles.VAS.c0/3*(u-mParams.muscles.VAS.qMx)^3
  pennation : Gain  Gain=mParams.muscles.HAB.rho
  pennation1 : Gain  Gain=mParams.muscles.HAD.rho
  pennation10 : Gain  Gain=mParams.muscles.GAS.rhoK
  pennation11 : Gain  Gain=mParams.muscles.GAS.rhoA
  pennation12 : Gain  Gain=mParams.muscles.SOL.rho
  pennation13 : Gain  Gain=mParams.muscles.TA.rho
  pennation2 : Gain  Gain=mParams.muscles.HFL.rho
  pennation3 : Gain  Gain=mParams.muscles.GLU.rho
  pennation4 : Gain  Gain=mParams.muscles.HAM.rhoH
  pennation5 : Gain  Gain=mParams.muscles.HAM.rhoK
  pennation6 : Gain  Gain=mParams.muscles.RF.rhoH
  pennation7 : Gain  Gain=mParams.muscles.RF.rhoK
  pennation8 : Gain  Gain=mParams.muscles.VAS.rho
  pennation9 : Gain  Gain=mParams.muscles.BFSH.rho
  reference length : Constant  Value=mParams.muscles.loptVec+mParams.muscles.lslackVec
  lmtc [m x11] : Outport  VectorParamsAs1DForOutWhenUnconnected=off
  wires:
  dl(q) for HAB/1 -> pennation/1
  dl(q) for HFL/1 -> pennation2/1
  dl(q) for HAM around knee/1 -> pennation5/1
  dl(q) for BFSH/1 -> pennation9/1
  dl(q) for HAM around hip/1 -> pennation4/1
  qAnkle [rad]/1 -> dl(q) for TA/1, dl(q) for SOL/1, dl(q) for GAS around ankle/1  "qA"
  dl(q) for TA/1 -> pennation13/1
  dl(q) for HAD/1 -> pennation1/1
  dl(q) for GLU/1 -> pennation3/1
  dl(q) for RF around knee/1 -> pennation7/1
  dl(q) for SOL/1 -> pennation12/1
  qHipPitch [rad]/1 -> dl(q) for HAM around hip/1, dl(q) for RF around hip/1, dl(q) for GLU/1, dl(q) for HFL/1  "qHP"
  dl(q) for RF around hip/1 -> pennation6/1
  qHipRoll [rad]/1 -> dl(q) for HAD/1, dl(q) for HAB/1  "qHR"
  Sum1/1 -> Mux/6
  qKnee [rad]/1 -> dl(q) for HAM around knee/1, dl(q) for VAS/1, dl(q) for GAS around knee/1, dl(q) for BFSH/1, dl(q) for RF around knee/1  "qK"
  Sum/1 -> Mux/5
  Sum2/1 -> Mux/9
  dl(q) for GAS around knee/1 -> pennation10/1
  dl(q) for GAS around ankle/1 -> pennation11/1
  dl(q) for VAS/1 -> pennation8/1
  Mux/1 -> Sum3/1  "dl"
  Sum3/1 -> lmtc [m x11]/1  "lmtc"
  reference length/1 -> Sum3/2  "lref"
  pennation/1 -> Mux/1
  pennation1/1 -> Mux/2
  pennation2/1 -> Mux/3
  pennation3/1 -> Mux/4
  pennation4/1 -> Sum/1
  pennation5/1 -> Sum/2
  pennation6/1 -> Sum1/1
  pennation7/1 -> Sum1/2
  pennation8/1 -> Mux/7
  pennation9/1 -> Mux/8
  pennation10/1 -> Sum2/1
  pennation11/1 -> Sum2/2
  pennation12/1 -> Mux/10
  pennation13/1 -> Mux/11

== system ramadan_2021/Muscle Actuation Layer/Muscles Left/Muscle Torque Contributions1 ==
  note: Leg Muscle Torque Contributions
  qKnee [rad] : Inport
  qAnkle [rad] : Inport  Port=2
  FmVec [N x11] : Inport  Port=3
  Demux1 : Demux  Outputs=11
  Product{1..6} (6 alike) : Product
  Subsystem : Subsystem
  Sum : Sum  Inputs=+-
  Sum1 : Sum  Inputs=-++-
  Sum2 : Sum  Inputs=-++--
  Sum3 : Sum  Inputs=++-
  r(q) RF around knee : Fcn  Expr=mParams.muscles.RF.rMxK - mParams.muscles.RF.c0K*(u-mParams.muscles.RF.qMxK)^2
  r(q) RGAS around ankle : Fcn  Expr=mParams.muscles.GAS.rMxA - mParams.muscles.GAS.c0A*(u-mParams.muscles.GAS.qMxA)^2
  r(q) RGAS around knee : Fcn  Expr=mParams.muscles.GAS.rMxK - mParams.muscles.GAS.c0K*(u-mParams.muscles.GAS.qMxK)^2
  r(q) RSOL : Fcn  Expr=mParams.muscles.SOL.rMx - mParams.muscles.SOL.c0*(u-mParams.muscles.SOL.qMx)^2
  r(q) RTA : Fcn  Expr=mParams.muscles.TA.rMx - mParams.muscles.TA.c0*(u-mParams.muscles.TA.qMx)^2
  r(q) for BFSH : Gain  Gain=mParams.muscles.BFSH.r0
  r(q) for GLU : Gain  Gain=mParams.muscles.GLU.r0
  r(q) for HAB : Gain  Gain=mParams.muscles.HAB.r0
  r(q) for HAD : Gain  Gain=mParams.muscles.HAD.r0
  r(q) for HAM at hip : Gain  Gain=mParams.muscles.HAM.r0H
  r(q) for HAM at knee : Gain  Gain=mParams.muscles.HAM.r0K
  r(q) for HFL : Gain  Gain=mParams.muscles.HFL.r0
  r(q) for RF : Gain  Gain=mParams.muscles.RF.r0H
  r(q) for VAS : Fcn  Expr=mParams.muscles.VAS.rMx - mParams.muscles.VAS.c0*(u-mParams.muscles.VAS.qMx)^2
  tauHP [Nm] : Outport  VectorParamsAs1DForOutWhenUnconnected=off
  tauHR [Nm] : Outport  Port=2  VectorParamsAs1DForOutWhenUnconnected=off
  tauK [Nm] : Outport  Port=3  VectorParamsAs1DForOutWhenUnconnected=off
  tauA [Nm] : Outport  Port=4  VectorParamsAs1DForOutWhenUnconnected=off
  Leg Torque : Outport  Port=5  VectorParamsAs1DForOutWhenUnconnected=off
  wires:
  qKnee [rad]/1 -> r(q) RGAS around knee/1, r(q) RF around knee/1, r(q) for VAS/1  "qK"
  qAnkle [rad]/1 -> r(q) RTA/1, r(q) RSOL/1, r(q) RGAS around ankle/1  "qA"
  FmVec [N x11]/1 -> Demux1/1
  Demux1/1 -> r(q) for HAB/1  "HAB"
  Demux1/2 -> r(q) for HAD/1  "HAD"
  r(q) for HAD/1 -> Sum/2
  r(q) for HAB/1 -> Sum/1
  Demux1/3 -> r(q) for HFL/1  "HFL"
  Demux1/4 -> r(q) for GLU/1  "GLU"
  Demux1/5 -> r(q) for HAM at knee/1, r(q) for HAM at hip/1  "HAM"
  Demux1/6 -> Product1/1, r(q) for RF/1  "RF"
  r(q) for RF/1 -> Sum1/4
  r(q) RF around knee/1 -> Product1/2
  Product1/1 -> Sum2/2
  r(q) for HAM at knee/1 -> Sum2/1
  r(q) for HAM at hip/1 -> Sum1/3
  r(q) for GLU/1 -> Sum1/2
  r(q) for HFL/1 -> Sum1/1
  Sum1/1 -> tauHP [Nm]/1
  Demux1/7 -> Subsystem/1(F VAS), Product2/1  "VAS"
  r(q) for VAS/1 -> Subsystem/2(Moment Arm VAS), Product2/2
  Demux1/8 -> r(q) for BFSH/1  "BFSH"
  Demux1/9 -> Product3/1, Product4/1  "GAS"
  r(q) RGAS around knee/1 -> Product3/2
  Product2/1 -> Sum2/3
  r(q) for BFSH/1 -> Sum2/4
  Product3/1 -> Sum2/5
  Sum2/1 -> tauK [Nm]/1
  r(q) RGAS around ankle/1 -> Product4/2
  r(q) RSOL/1 -> Product5/2, Subsystem/4(Moment Arm SOL)
  Demux1/10 -> Subsystem/3(F SOL), Product5/1  "SOL"
  r(q) RTA/1 -> Product6/2
  Demux1/11 -> Product6/1  "TA"
  Product4/1 -> Sum3/1
  Product5/1 -> Sum3/2
  Product6/1 -> Sum3/3
  Sum3/1 -> tauA [Nm]/1
  Sum/1 -> tauHR [Nm]/1
  Subsystem/1("Leg Torque ") -> Leg Torque/1

== system ramadan_2021/Muscle Actuation Layer/Muscles Right/Muscle Dynamics (Vectorized) ==
  note: Excitation Contraction Coupling
  lmtc [m] : Inport
  STIM : Inport  Port=2
  1 : Product  Inputs=**  InputSameDT=on  SaturateOnIntegerOverflow=on  OutDataTypeStr=Inherit: Same as first input
  1./lopt : Gain  Gain=1./mParams.muscles.loptVec  SaturateOnIntegerOverflow=on  OutDataTypeStr=Inherit: Same as input  ParamDataTypeStr=Inherit: Same as input
  1./lopt2 : Gain  Gain=1/mParams.muscles.tauA  SaturateOnIntegerOverflow=on  OutDataTypeStr=Inherit: Same as input  ParamDataTypeStr=Inherit: Same as input
  1/lslack : Gain  Gain=1./mParams.muscles.lslackVec  SaturateOnIntegerOverflow=on  OutDataTypeStr=Inherit: Same as input  ParamDataTypeStr=Inherit: Same as input
  BE force-length relation : Subsystem
  CE force-length relation : Subsystem
  CE inverse force-velocity relation : Subsystem
  Constant : Constant  Value=mParams.muscles.lslackVec
  Fmax : Gain  Gain=mParams.muscles.FmaxVec  SaturateOnIntegerOverflow=on  OutDataTypeStr=Inherit: Same as input  ParamDataTypeStr=Inherit: Same as input
  Fv = Fse / (A*Fce) : Product  Inputs=*/  InputSameDT=on  SaturateOnIntegerOverflow=on  OutDataTypeStr=Inherit: Same as first input
  Integrator : Integrator  InitialConditionSource=external  LowerSaturationLimit=0.05
  Integrator1 : Integrator  InitialConditionSource=external  LowerSaturationLimit=0.05
  PE force-length relation : Subsystem
  SE force-length relation : Subsystem
  Sum : Sum  Inputs=|+-  InputSameDT=on  SaturateOnIntegerOverflow=on  OutDataTypeStr=Inherit: Same as first input
  Sum1 : Sum  Inputs=|+-  InputSameDT=on  SaturateOnIntegerOverflow=on  OutDataTypeStr=Inherit: Same as first input
  Sum2 : Sum  Inputs=|-+  InputSameDT=on  SaturateOnIntegerOverflow=on  OutDataTypeStr=Inherit: Same as first input
  Sum3 : Sum  Inputs=+++  InputSameDT=on  SaturateOnIntegerOverflow=on  OutDataTypeStr=Inherit: Same as first input
  Sum4 : Sum  InputSameDT=on  SaturateOnIntegerOverflow=on  OutDataTypeStr=Inherit: Same as first input
  avoid div by 0 : Constant  Value=eps
  preA : Constant  Value=mParams.muscles.preA
  vmax*lopt : Gain  Gain=mParams.muscles.vmaxVec  SaturateOnIntegerOverflow=on  OutDataTypeStr=Inherit: Same as input  ParamDataTypeStr=Inherit: Same as input
  Fmtc : Outport  InitialOutput=0  VectorParamsAs1DForOutWhenUnconnected=off
  Lce : Outport  Port=2  InitialOutput=0  VectorParamsAs1DForOutWhenUnconnected=off
  Vce : Outport  Port=3  InitialOutput=0  VectorParamsAs1DForOutWhenUnconnected=off
  A : Outport  Port=4  InitialOutput=0  VectorParamsAs1DForOutWhenUnconnected=off
  ForceLengthFactor : Outport  Port=5  VectorParamsAs1DForOutWhenUnconnected=off
  tag scope: fl_R=global, fv_R=global
  wires:
  1./lopt2/1 -> Integrator1/1
  Sum1/1 -> 1./lopt2/1
  CE inverse force-velocity relation/1(v[vmax]) -> vmax*lopt/1
  Fv = Fse / (A*Fce)/1 -> CE inverse force-velocity relation/1(Fv[Fmax]), [fv_R]  "fv"
  Sum3/1 -> Fv = Fse / (A*Fce)/2
  Sum4/1 -> Fv = Fse / (A*Fce)/1
  SE force-length relation/1(fse [Fmax]) -> Fmax/1, Sum4/1
  STIM/1 -> Sum1/1
  Integrator1/1 -> Sum1/2, A/1, 1/2
  1/lslack/1 -> SE force-length relation/1(lse [lslack])
  Fmax/1 -> Fmtc/1  "Fmtc"
  lmtc [m]/1 -> Sum2/2, Sum/1  "lmtc"
  vmax*lopt/1 -> Vce/1, Integrator/1  "vce"
  1./lopt/1 -> CE force-length relation/1(lce [lopt]), PE force-length relation/1(lce [lopt]), BE force-length relation/1(lce [lopt])
  Integrator/1 -> Lce/1, 1./lopt/1, Sum/2  "lce"
  1/1 -> Sum3/3
  avoid div by 0/1 -> Sum3/2
  Sum2/1 -> Integrator/2
  Sum/1 -> 1/lslack/1  "lse"
  Constant/1 -> Sum2/1
  PE force-length relation/1(fpe [Fmax]) -> Sum3/1
  BE force-length relation/1(fbe [Fmax]) -> Sum4/2
  preA/1 -> Integrator1/2
  CE force-length relation/1(fce [Fmax]) -> [fl_R], ForceLengthFactor/1, 1/1

== system ramadan_2021/Muscle Actuation Layer/Muscles Right/Muscle Length Vector ==
  note: Muscle Length Vector
  qHipPitch [rad] : Inport
  qHipRoll [rad] : Inport  Port=2
  qKnee [rad] : Inport  Port=3
  qAnkle [rad] : Inport  Port=4
  Mux : Mux  Inputs=11
  Sum : Sum  Inputs=-+
  Sum1 : Sum  Inputs=+-
  Sum2 : Sum  Inputs=+-
  Sum3 : Sum  Inputs=|++
  dl(q) for BFSH : Fcn  Expr=mParams.muscles.BFSH.r0 *(u-mParams.muscles.BFSH.qRef)
  dl(q) for GAS around ankle : Fcn  Expr=mParams.muscles.GAS.c1A + mParams.muscles.GAS.rMxA*u - mParams.muscles.GAS.c0A/3*(u-mParams.muscles.GAS.qMxA)^3
  dl(q) for GAS around knee : Fcn  Expr=mParams.muscles.GAS.c1K + mParams.muscles.GAS.rMxK*u - mParams.muscles.GAS.c0K/3*(u-mParams.muscles.GAS.qMxK)^3
  dl(q) for GLU : Fcn  Expr=-mParams.muscles.GLU.r0 *(u-mParams.muscles.GLU.qRef)
  dl(q) for HAB : Fcn  Expr=-mParams.muscles.HAB.r0 *(u-mParams.muscles.HAB.qRef)
  dl(q) for HAD : Fcn  Expr=mParams.muscles.HAD.r0 *(u-mParams.muscles.HAD.qRef)
  dl(q) for HAM around hip : Fcn  Expr=mParams.muscles.HAM.r0H *(u-mParams.muscles.HAM.qRefH)
  dl(q) for HAM around knee : Fcn  Expr=mParams.muscles.HAM.r0K *(u-mParams.muscles.HAM.qRefK)
  dl(q) for HFL : Fcn  Expr=mParams.muscles.HFL.r0 *(u-mParams.muscles.HFL.qRef)
  dl(q) for RF around hip : Fcn  Expr=mParams.muscles.RF.r0H *(u-mParams.muscles.RF.qRefH)
  dl(q) for RF around knee : Fcn  Expr=mParams.muscles.RF.c1K + mParams.muscles.RF.rMxK*u - mParams.muscles.RF.c0K/3*(u-mParams.muscles.RF.qMxK)^3
  dl(q) for SOL : Fcn  Expr=-mParams.muscles.SOL.c1 - mParams.muscles.SOL.rMx*u + mParams.muscles.SOL.c0/3*(u-mParams.muscles.SOL.qMx)^3
  dl(q) for TA : Fcn  Expr=mParams.muscles.TA.c1 + mParams.muscles.TA.rMx*u - mParams.muscles.TA.c0/3*(u-mParams.muscles.TA.qMx)^3
  dl(q) for VAS : Fcn  Expr=-mParams.muscles.VAS.c1 - mParams.muscles.VAS.rMx*u + mParams.muscles.VAS.c0/3*(u-mParams.muscles.VAS.qMx)^3
  pennation : Gain  Gain=mParams.muscles.HAB.rho
  pennation1 : Gain  Gain=mParams.muscles.HAD.rho
  pennation10 : Gain  Gain=mParams.muscles.GAS.rhoK
  pennation11 : Gain  Gain=mParams.muscles.GAS.rhoA
  pennation12 : Gain  Gain=mParams.muscles.SOL.rho
  pennation13 : Gain  Gain=mParams.muscles.TA.rho
  pennation2 : Gain  Gain=mParams.muscles.HFL.rho
  pennation3 : Gain  Gain=mParams.muscles.GLU.rho
  pennation4 : Gain  Gain=mParams.muscles.HAM.rhoH
  pennation5 : Gain  Gain=mParams.muscles.HAM.rhoK
  pennation6 : Gain  Gain=mParams.muscles.RF.rhoH
  pennation7 : Gain  Gain=mParams.muscles.RF.rhoK
  pennation8 : Gain  Gain=mParams.muscles.VAS.rho
  pennation9 : Gain  Gain=mParams.muscles.BFSH.rho
  reference length : Constant  Value=mParams.muscles.loptVec+mParams.muscles.lslackVec
  lmtc [m x11] : Outport  VectorParamsAs1DForOutWhenUnconnected=off
  wires:
  dl(q) for HAB/1 -> pennation/1
  dl(q) for HFL/1 -> pennation2/1
  dl(q) for HAM around knee/1 -> pennation5/1
  dl(q) for BFSH/1 -> pennation9/1
  dl(q) for HAM around hip/1 -> pennation4/1
  qAnkle [rad]/1 -> dl(q) for TA/1, dl(q) for SOL/1, dl(q) for GAS around ankle/1  "qA"
  dl(q) for TA/1 -> pennation13/1
  dl(q) for HAD/1 -> pennation1/1
  dl(q) for GLU/1 -> pennation3/1
  dl(q) for RF around knee/1 -> pennation7/1
  dl(q) for SOL/1 -> pennation12/1
  qHipPitch [rad]/1 -> dl(q) for HAM around hip/1, dl(q) for RF around hip/1, dl(q) for GLU/1, dl(q) for HFL/1  "qHP"
  dl(q) for RF around hip/1 -> pennation6/1
  qHipRoll [rad]/1 -> dl(q) for HAD/1, dl(q) for HAB/1  "qHR"
  Sum1/1 -> Mux/6
  qKnee [rad]/1 -> dl(q) for HAM around knee/1, dl(q) for VAS/1, dl(q) for GAS around knee/1, dl(q) for BFSH/1, dl(q) for RF around knee/1  "qK"
  Sum/1 -> Mux/5
  Sum2/1 -> Mux/9
  dl(q) for GAS around knee/1 -> pennation10/1
  dl(q) for GAS around ankle/1 -> pennation11/1
  dl(q) for VAS/1 -> pennation8/1
  Mux/1 -> Sum3/1  "dl"
  Sum3/1 -> lmtc [m x11]/1  "lmtc"
  reference length/1 -> Sum3/2  "lref"
  pennation2/1 -> Mux/3
  pennation3/1 -> Mux/4
  pennation4/1 -> Sum/1
  pennation5/1 -> Sum/2
  pennation6/1 -> Sum1/1
  pennation7/1 -> Sum1/2
  pennation8/1 -> Mux/7
  pennation9/1 -> Mux/8
  pennation10/1 -> Sum2/1
  pennation11/1 -> Sum2/2
  pennation12/1 -> Mux/10
  pennation13/1 -> Mux/11
  pennation/1 -> Mux/1
  pennation1/1 -> Mux/2
